simulink model "AnalogControl"  (R2024a)
settings: Solver=VariableStepAuto  StartTime=0.0  StopTime=10.0  MaxStep=0.1  RelTol=1e-3  EnableMultiTasking=on
undefined symbols (not defined in the file): Ka, Kf, Ki, Kq, Tal, Ts, W1, W2
libraries: simulink x1
settings Model: DataDictionary=controller.sldd  EnableAccessToBaseWorkspace=off  Creator=The MathWorks, Inc.
settings SolverCC: AlgebraicLoopSolver=TrustRegion
settings DataIOCC: LimitDataPoints=on  SaveFormat=Array  SaveOutput=off  SignalLogging=off  SaveTime=off  ReturnWorkspaceOutputs=off  SignalLoggingName=AnalogControl
settings OptimizationCC: DefaultParameterBehavior=Inlined  ReuseModelBlockBuffer=off  ExpressionDepthLimit=2147483647  InitFltsAndDblsToZero=on  LifeSpan=inf
settings DebuggingCC: SaveWithParameterizedLinksMsg=none  UnderspecifiedInitializationDetection=Classic  MergeDetectMultiDrivingBlocksExec=none  SignalResolutionControl=TryResolveAllWithWarning  SolverPrmCheckMsg=warning  MultiTaskDSMMsg=warning  MultiTaskCondExecSysMsg=none  FcnCallInpInsideContextMsg=warning  UnconnectedInputMsg=warning  UnconnectedOutputMsg=warning  UnconnectedLineMsg=warning  AllowSymbolicDim=off  StateNameClashWarn=warning  SFUnexpectedBacktrackingDiag=warning  SFNoUnconditionalDefaultTransitionDiag=warning  SFExecutionAtInitializationDiag=none  ArithmeticOperatorsInVariantConditions=warning
settings HardwareCC: ProdBitPerPointer=32  ProdLargestAtomicFloat=None  ProdIntDivRoundTo=Undefined  ProdEndianess=Unspecified  ProdWordSize=32  ProdHWDeviceType=32-bit Generic
settings ModelReferenceCC: EnableRefExpFcnMdlSchedulingChecks=on  PropagateSignalLabelsOutOfModel=off
settings SFSimCC: SimUseLocalCustomCode=off  CustomCodeUndefinedFunction=UseInterfaceOnly
settings RTWCC: RTWUseLocalCustomCode=off  GPUComputeCapability=3.5
settings CodeAppCC: StateflowObjectComments=on
settings GRTTargetCC: TargetFcnLib=ansi_tfl_tmw.mat  TargetLangStandard=C89/C90 (ANSI)  CombineOutputUpdateFcns=off  GRTInterface=on
settings ConfigComp: CovMetricSettings=dw  CovSaveCumulativeToWorkspaceVar=on  CovSaveSingleToWorkspaceVar=on  CovExternalEMLEnable=off  CovSFcnEnable=off

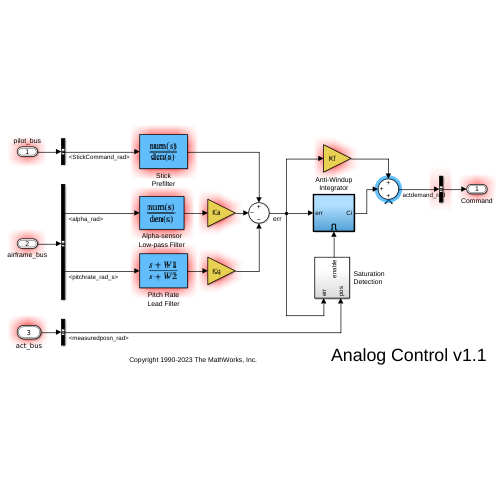
[thumbnail: Simulink's stored preview of the top-level diagram]
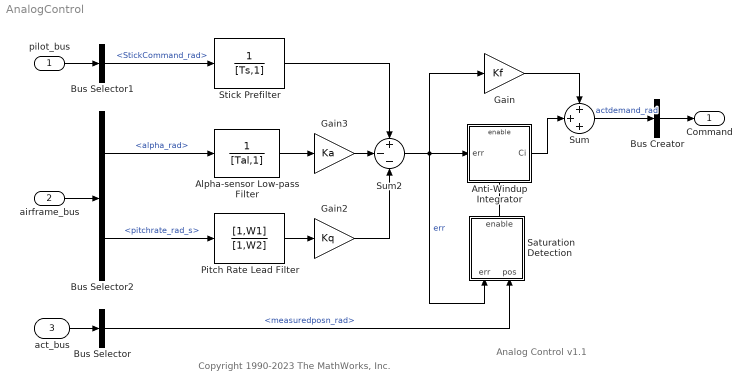
== system AnalogControl ==
  note: Analog Control v1.1
  note: Copyright 1990-2023 The MathWorks, Inc.
  pilot_bus : Inport  OutDataTypeStr=Bus: PILOT_BUS
  airframe_bus : Inport  Port=2  OutDataTypeStr=Bus: AIRFRAME_BUS
  act_bus : Inport  Port=3  OutDataTypeStr=Bus: ACT_BUS
  Alpha-sensor Low-pass Filter : TransferFcn  Denominator=[Tal,1]
  Anti-Windup Integrator : Subsystem  TreatAsAtomicUnit=on
      settings: RTWSystemCode=Inline
  Bus Creator : BusCreator  Inputs=1  OutDataTypeStr=Bus: CONTROL_BUS
  Bus Selector : BusSelector  OutputSignals=measuredposn_rad
  Bus Selector1 : BusSelector  OutputSignals=StickCommand_rad
  Bus Selector2 : BusSelector  OutputSignals=alpha_rad,pitchrate_rad_s
  Gain : Gain  Gain=Kf  SaturateOnIntegerOverflow=on  OutDataTypeStr=Inherit: Same as input  ParamDataTypeStr=Inherit: Same as input
  Gain2 : Gain  Gain=Kq  SaturateOnIntegerOverflow=on  OutDataTypeStr=Inherit: Same as input  ParamDataTypeStr=Inherit: Same as input
  Gain3 : Gain  Gain=Ka  SaturateOnIntegerOverflow=on  OutDataTypeStr=Inherit: Same as input  ParamDataTypeStr=Inherit: Same as input
  Pitch Rate Lead Filter : TransferFcn  Numerator=[1,W1]  Denominator=[1,W2]
  Saturation Detection : Subsystem
  Stick Prefilter : TransferFcn  Denominator=[Ts,1]
  Sum : Sum  Inputs=3  InputSameDT=on  SaturateOnIntegerOverflow=on  OutDataTypeStr=Inherit: Same as first input
  Sum2 : Sum  Inputs=+--  InputSameDT=on  SaturateOnIntegerOverflow=on  OutDataTypeStr=Inherit: Same as first input
  Command : Outport  OutDataTypeStr=Bus: CONTROL_BUS  VectorParamsAs1DForOutWhenUnconnected=off
  wires:
  Saturation Detection/1(enable) -> Anti-Windup Integrator/Enable
  Bus Selector/1 -> Saturation Detection/2(pos)  "<measuredposn_rad>"
  Bus Selector2/2 -> Pitch Rate Lead Filter/1  "<pitchrate_rad_s>"
  Bus Selector2/1 -> Alpha-sensor Low-pass Filter/1  "<alpha_rad>"
  Gain/1 -> Sum/1
  Gain3/1 -> Sum2/2
  Pitch Rate Lead Filter/1 -> Gain2/1
  Stick Prefilter/1 -> Sum2/1
  Gain2/1 -> Sum2/3
  Alpha-sensor Low-pass Filter/1 -> Gain3/1
  Bus Selector1/1 -> Stick Prefilter/1  "<StickCommand_rad>"
  Anti-Windup Integrator/1(Ci) -> Sum/2
  Sum2/1 -> Saturation Detection/1(err), Anti-Windup Integrator/1(err), Gain/1  "err"
  pilot_bus/1 -> Bus Selector1/1
  act_bus/1 -> Bus Selector/1
  airframe_bus/1 -> Bus Selector2/1
  Sum/1 -> Bus Creator/1  "actdemand_rad"
  Bus Creator/1 -> Command/1

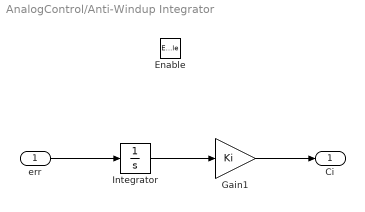
== system AnalogControl/Anti-Windup Integrator ==
  err : Inport
  Enable : EnablePort
  Gain1 : Gain  Gain=Ki  SaturateOnIntegerOverflow=on  OutDataTypeStr=Inherit: Same as input  ParamDataTypeStr=Inherit: Same as input
  Integrator : Integrator
  Ci : Outport  InitialOutput=0  VectorParamsAs1DForOutWhenUnconnected=off
  wires:
  Gain1/1 -> Ci/1
  Integrator/1 -> Gain1/1
  err/1 -> Integrator/1

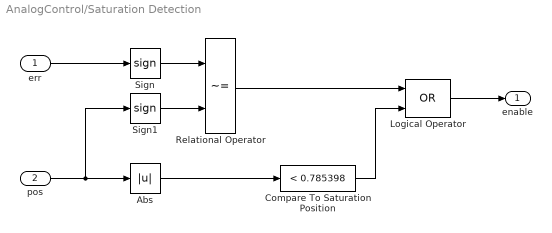
== system AnalogControl/Saturation Detection ==
  err : Inport
  pos : Inport  Port=2
  Abs : Abs  ZeroCross=off  SaturateOnIntegerOverflow=off
  Compare To Saturation Position : simulink/Logic and Bit Operations/Compare To Constant  relop=<  const=0.785398  OutDataTypeStr=boolean  ZeroCross=off
  Logical Operator : Logic  Operator=OR  AllPortsSameDT=off  OutDataTypeStr=boolean
  Relational Operator : RelationalOperator  Operator=~=  OutDataTypeStr=boolean  ZeroCross=off  InputSameDT=off
  Sign : Signum  ZeroCross=off
  Sign1 : Signum  ZeroCross=off
  enable : Outport  VectorParamsAs1DForOutWhenUnconnected=off
  wires:
  Logical Operator/1 -> enable/1
  err/1 -> Sign/1
  Abs/1 -> Compare To Saturation Position/1
  Sign1/1 -> Relational Operator/2
  Compare To Saturation Position/1 -> Logical Operator/2
  Relational Operator/1 -> Logical Operator/1
  Sign/1 -> Relational Operator/1
  pos/1 -> Abs/1, Sign1/1
